simulink model "springblock2dof"  (R2017b)
settings: Solver=VariableStepAuto  StartTime=0.0  StopTime=100.0  RelTol=1e-3
values from neighbouring files (symbols this model uses):
  d1 = xlsread('d.xlsx')    [model_edited2.m]
  F = @(x) (exp(x/c) + exp(-x/c))/2    [LAB10.m]    (also in LUdecomp.m = [0;0;-P]; Lab7.m = @(x) [x(1) + x(2) - 2; x(1)*x(3) + x(4)*x(2); x(1)*x(3)^2 + ; Lab8.m = 100000; Stress_fem.m = [-12e03; -8e03])
  m1 = 1e4    (= 10000)    [Burgerseqn1d.m]    (also in LAB10.m)
  m2 = 9e3    (= 9000)    [Burgerseqn1d.m]    (also in LAB10.m)
undefined symbols (not defined in the file or in its folder): d2, k1, k2
settings Model: Creator=OCAC  LastModifiedBy=OCAC

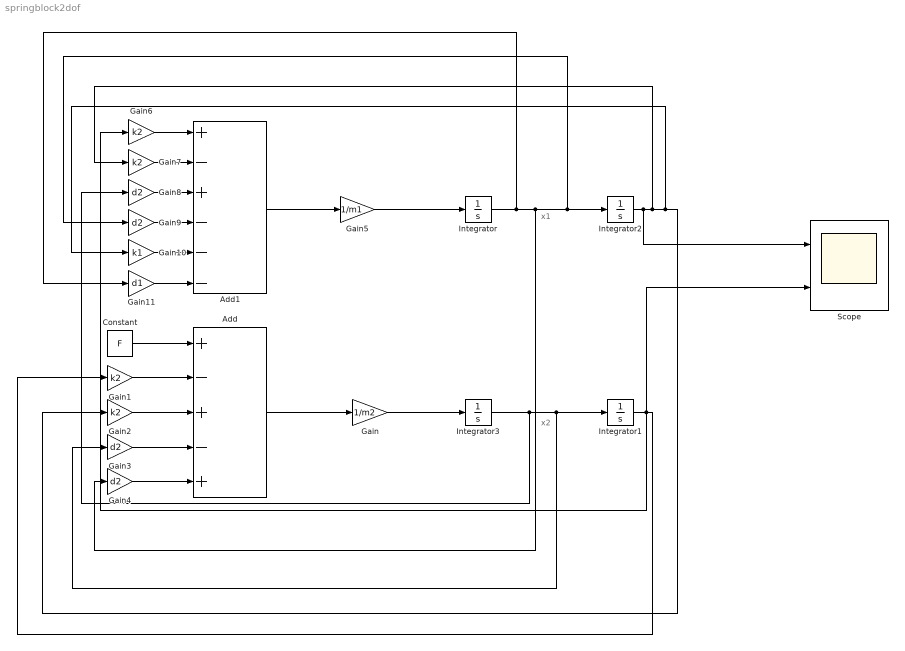
== system springblock2dof ==
  note: x2
  note: x1
  Add : Sum  Inputs=+-+-+
  Add1 : Sum  Inputs=+-+---
  Constant : Constant  Value=F
  Gain : Gain  Gain=1/m2
  Gain{1..2,6..7} (4 alike) : Gain  Gain=k2
  Gain10 : Gain  Gain=k1
  Gain11 : Gain  Gain=d1
  Gain{3..4,8..9} (4 alike) : Gain  Gain=d2
  Gain5 : Gain  Gain=1/m1
  Integrator{,1..3} (4 alike) : Integrator
  Scope : Scope  NumInputPorts=2
  wires:
  Integrator/1 -> Gain11/1, Gain4/1, Gain9/1, Integrator2/1
  Integrator3/1 -> Gain8/1, Gain3/1, Integrator1/1
  Add/1 -> Gain/1
  Gain/1 -> Integrator3/1
  Constant/1 -> Add/1
  Gain1/1 -> Add/2
  Gain2/1 -> Add/3
  Integrator1/1 -> Scope/2, Gain6/1, Gain1/1
  Integrator2/1 -> Scope/1, Gain7/1, Gain10/1, Gain2/1
  Gain3/1 -> Add/4
  Gain4/1 -> Add/5
  Gain5/1 -> Integrator/1
  Add1/1 -> Gain5/1
  Gain6/1 -> Add1/1
  Gain7/1 -> Add1/2
  Gain8/1 -> Add1/3
  Gain9/1 -> Add1/4
  Gain10/1 -> Add1/5
  Gain11/1 -> Add1/6
